simulink model "untitled1"  (R2023a)
settings: Solver=VariableStepAuto  StartTime=0.0  StopTime=10.0  RelTol=1e-3
values from neighbouring files (symbols this model uses):
  Ap = 3.35e-4    (= 0.000335)    [Main.m]    (also in SweepTest.m; myActiveSuspensions.mat)
  g = 9.81    [Main.m]    (also in SweepTest.m; myActiveSuspensions.mat)
settings Model: Creator=aleze  LastModifiedBy=aleze

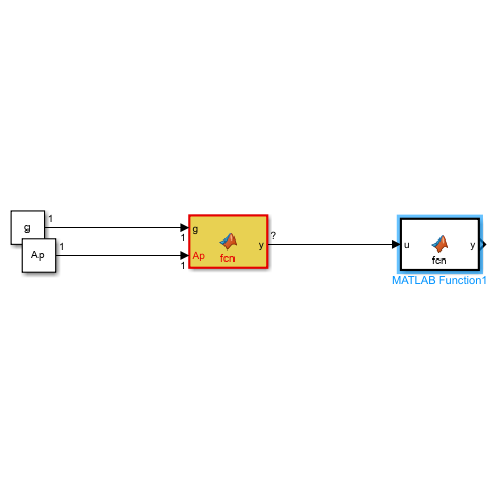
[thumbnail: Simulink's stored preview of the top-level diagram]
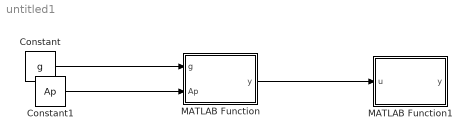
== system untitled1 ==
  Constant : Constant  Value=g
  Constant1 : Constant  Value=Ap
  MATLAB Function : MATLAB Function  TreatAsAtomicUnit=on
  MATLAB Function1 : MATLAB Function  TreatAsAtomicUnit=on
  wires:
  MATLAB Function/1(y) -> MATLAB Function1/1(u)
  Constant1/1 -> MATLAB Function/2(Ap)
  Constant/1 -> MATLAB Function/1(g)

== matlab function untitled1/MATLAB Function ==
  data: g input; y output; Ap input
function y = fcn(g,Ap)
myAs.g = g;
myAs.Ap = Ap;
y = myAs;
end

== matlab function untitled1/MATLAB Function1 ==
  data: u input; y output
function y = fcn(u)

y = u.g;
